simulink model "Main"  (R2021a)
settings: Solver=ode4  StartTime=0.0  StopTime=param.taskDuration  FixedStep=0.005  RelTol=1e-3
InitFcn:
  | Init
StopFcn:
  | StopSim
values from neighbouring files (symbols this model uses):
  jaco = Jaco2(samplingNumber,vrepInstance)    [Init.m]
undefined symbols (not defined in the file or in its folder): DiscIntNeverNeededParam, param
settings Model: EnablePacing=on  Creator=dell  LastModifiedBy=dell

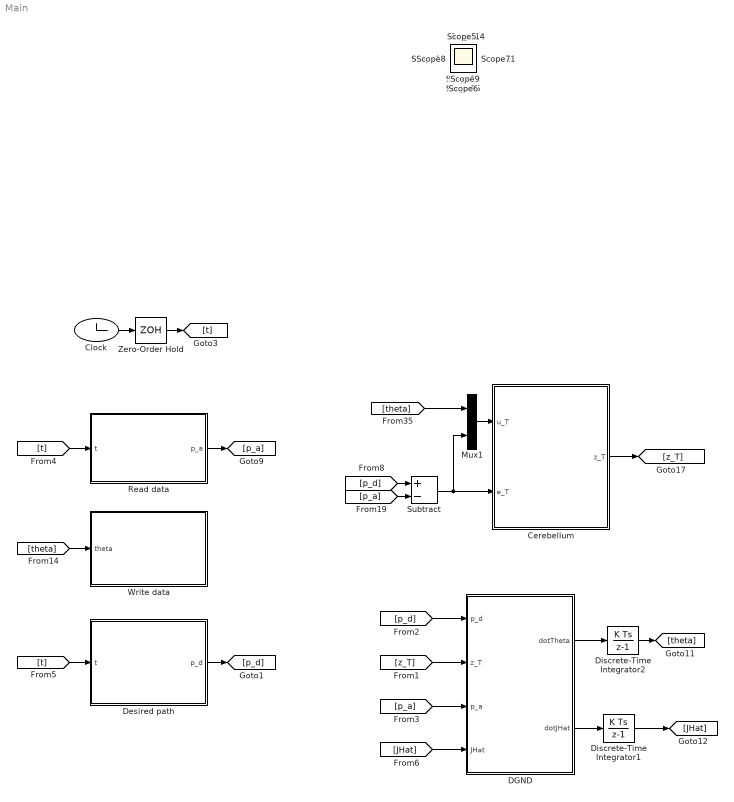
== system Main ==
  Cerebellum : MATLAB Function  TreatAsAtomicUnit=on
  Clock : Clock
  DGND : MATLAB Function  TreatAsAtomicUnit=on
  Desired path : MATLAB Function  TreatAsAtomicUnit=on
  Discrete-Time Integrator1 : DiscreteIntegrator  InitialCondition=jaco.JHat(:,:,1)  SampleTime=-1  OutDataTypeStr=double  ICPrevOutput=DiscIntNeverNeededParam  ICPrevScaledInput=DiscIntNeverNeededParam
  Discrete-Time Integrator2 : DiscreteIntegrator  InitialCondition=jaco.theta(:,1)  SampleTime=-1  OutDataTypeStr=double  ICPrevOutput=DiscIntNeverNeededParam  ICPrevScaledInput=DiscIntNeverNeededParam
  Mux1 : Mux  Inputs=2
  Read data : MATLAB Function  TreatAsAtomicUnit=on
  Subtract : Sum  Inputs=+-
  Write data : MATLAB Function  TreatAsAtomicUnit=on
  Zero-Order Hold : ZeroOrderHold  SampleTime=param.samplingGap
  Scope{,1..15} (16 alike) : Scope
  wires:
  Clock/1 -> Zero-Order Hold/1
  Zero-Order Hold/1 -> [t]
  [t] -> Read data/1(t)
  [t] -> Desired path/1(t)
  [theta] -> Write data/1(theta)
  Discrete-Time Integrator2/1 -> [theta]
  DGND/2(dotJHat) -> Discrete-Time Integrator1/1
  Discrete-Time Integrator1/1 -> [JHat]
  Read data/1(p_a) -> [p_a]
  [p_d] -> Subtract/1
  [p_a] -> Subtract/2
  Mux1/1 -> Cerebellum/1(u_T)
  Cerebellum/1(z_T) -> [z_T]
  [theta] -> Mux1/1
  Subtract/1 -> Mux1/2, Cerebellum/2(e_T)
  Desired path/1(p_d) -> [p_d]
  [z_T] -> DGND/2(z_T)
  [p_d] -> DGND/1(p_d)
  [p_a] -> DGND/3(p_a)
  [JHat] -> DGND/4(JHat)
  DGND/1(dotTheta) -> Discrete-Time Integrator2/1

== matlab function Main/Read data ==
  data: t input; p_a output
function p_a  = VREPRead(t)

coder.extrinsic('VrepRead');

p_a = zeros(7,1);
% theta = zeros(6,1);

output = double(VrepRead());

p_a = output(1:7);
% theta = output(8:13);

== matlab function Main/Write data ==
  data: theta input
function VREPWrite(theta)

coder.extrinsic('VrepWrite');
% To keep the robot stationary when Simulink begins to execute
% if t>0
    VrepWrite(theta)
% end

== matlab function Main/DGND ==
  data: p_d input; z_T input; p_a input; JHat input; dotTheta output; dotJHat output
function [dotTheta, dotJHat]   = DGND(p_d, z_T, p_a, JHat)
coder.extrinsic('DGND');
dotTheta = zeros(6,1);
dotJHat = zeros(7,6);

output = double(DGND(p_d, z_T, p_a, JHat));
dotTheta = output(1:6);
dotJHat = reshape(output(7:48), [7,6]);

== matlab function Main/Desired path ==
  data: t input; p_d output
function p_d = Path_Gnrt(t)
%#codegen

coder.extrinsic('PathGnrt');
p_d = zeros(7,1);
output = double(PathGnrt(t));
p_d = output(1:7);

== matlab function Main/Cerebellum ==
  data: u_T input; z_T output; e_T input
function z_T  = Cereb_Net(u_T, e_T)
coder.extrinsic('CerebNet');

z_T = zeros(7,1);
output = double(CerebNet(u_T, e_T));
z_T = output;
